simulink model "Model"  (R2024b)
settings: Solver=VariableStepAuto  StartTime=0.0  StopTime=20  RelTol=1e-2
values from neighbouring files (symbols this model uses):
  camber = 1 *pi/180    (= 0.0174532925199)    [var.m]
  cgToRearAxle = 0.7    [var.m]
  cgVerticalToAxlePlane = 0.1    [var.m]
  lammux = 0.65    [var.m]
  lammuy = 0.65    [var.m]
  mass = 200    [var.m]
  maxBrakePressure = 5000000    [var.m]
  tirePressure = 83000    [var.m]
  tireRadius = 0.2057    [var.m]
  trackWidth = 1    [var.m]
  wheelAngleLimit = 45 *pi/180    (= 0.785398163397)    [var.m]
  yawPolarInertia = 200    [var.m]
undefined symbols (not defined in the file or in its folder): SteerLim, Ts, VEH
libraries: sim3dlib x4, autolibsharedcoupling x2, sim3dautolib x2, vehdynlibviscommon x2, simulink x1, autolibshared x1, autolibshareddiff x1, autolibmappedmotor x1, vehdynlibdriver x1, vehdynlibsteering x1, vehdynlibtire x1, vehdynlibsuspension x1
(part 3 of 3)

== system Model/Visualization/3D Visualization/Enabled/3D Visualization/Ground Following/Annotations/Enabled/Determine Angles In UE Vehicle Body Frame ==
  WheelYaw : Inport
  Fx : Inport  Port=2
  Fy : Inport  Port=3
  Add : Sum
  Add1 : Sum
  Constant1 : Constant  Value=0
  Constant11 : Constant  Value=[zeros(4,1)]
  Constant12 : Constant  Value=[zeros(4,1); ones(4,1).*pi/2]
  Constant2 : Constant  Value=pi
  Constant3 : Constant  Value=[zeros(8,2)]
  Constant4 : Constant  Value=[zeros(12,2)]
  Constant6 : Constant  Value=repmat([0 pi/2 0],[4,1])
  Matrix Concatenate : Concatenate  Mode=Multidimensional array
  Matrix Concatenate1 : Concatenate  Mode=Multidimensional array  ConcatenateDimension=2
  Matrix Concatenate2 : Concatenate  Mode=Multidimensional array
  Matrix Concatenate3 : Concatenate  NumInputs=3  Mode=Multidimensional array
  Matrix Concatenate4 : Concatenate  Mode=Multidimensional array  ConcatenateDimension=2
  Switch8 : Switch  ZeroCross=off  SaturateOnIntegerOverflow=off  InputSameDT=off
  Rotation : Outport
  wires:
  Constant2/1 -> Switch8/1
  Matrix Concatenate2/1 -> Switch8/2
  Constant1/1 -> Switch8/3
  Constant3/1 -> Matrix Concatenate1/1
  Matrix Concatenate1/1 -> Matrix Concatenate/1
  Switch8/1 -> Add/1
  Constant6/1 -> Matrix Concatenate/2
  Fx/1 -> Matrix Concatenate2/1
  Fy/1 -> Matrix Concatenate2/2
  Add/1 -> Matrix Concatenate1/2
  Constant12/1 -> Add/2
  Constant11/1 -> Matrix Concatenate3/3
  WheelYaw/1 -> Matrix Concatenate3/1, Matrix Concatenate3/2
  Constant4/1 -> Matrix Concatenate4/1
  Matrix Concatenate3/1 -> Matrix Concatenate4/2
  Matrix Concatenate4/1 -> Add1/2
  Matrix Concatenate/1 -> Add1/1
  Add1/1 -> Rotation/1

== system Model/Visualization/3D Visualization/Enabled/3D Visualization/Physical Vehicle/Annotations/Enabled/Convert to string ==
  xdot : Inport
  MotorSpeed : Inport  Port=2
  Gear : Inport  Port=3
  Round : Rounding  Operator=round
  Round1 : Rounding  Operator=round
  Signal Specification : SignalSpecification  Unit=rpm
  Signal Specification1 : SignalSpecification  Unit=km/h
  String Concatenate1 : StringConcatenate  Inputs=3
  String Concatenate2 : StringConcatenate
  String Concatenate3 : StringConcatenate
  String Constant3 : StringConstant  String="\" km/h\\n\""
  String Constant4 : StringConstant  String="\" RPM\\n\""
  To String1 : ToString
  To String2 : ToString
  To String3 : ToString
  Unit Conversion : UnitConversion
  Unit Conversion1 : UnitConversion
  String : Outport
  wires:
  MotorSpeed/1 -> Unit Conversion/1
  Signal Specification/1 -> Round1/1
  String Constant4/1 -> String Concatenate3/2
  Signal Specification1/1 -> Round/1
  String Concatenate2/1 -> String Concatenate1/1
  To String2/1 -> String Concatenate2/1
  String Constant3/1 -> String Concatenate2/2
  To String1/1 -> String Concatenate1/3
  String Concatenate3/1 -> String Concatenate1/2
  To String3/1 -> String Concatenate3/1
  Round/1 -> To String2/1
  Round1/1 -> To String3/1
  String Concatenate1/1 -> String/1
  Gear/1 -> To String1/1
  Unit Conversion/1 -> Signal Specification/1
  Unit Conversion1/1 -> Signal Specification1/1
  xdot/1 -> Unit Conversion1/1

== system Model/Visualization/3D Visualization/Enabled/3D Visualization/Physical Vehicle/Annotations/Enabled/Determine Angles In UE Vehicle Body Frame ==
  WheelYaw : Inport
  Fx : Inport  Port=2
  Fy : Inport  Port=3
  Add : Sum
  Add1 : Sum
  Constant1 : Constant  Value=0
  Constant11 : Constant  Value=[zeros(4,1)]
  Constant12 : Constant  Value=[zeros(4,1); ones(4,1).*pi/2]
  Constant2 : Constant  Value=pi
  Constant3 : Constant  Value=[zeros(8,2)]
  Constant4 : Constant  Value=[zeros(12,2)]
  Constant6 : Constant  Value=repmat([0 pi/2 0],[4,1])
  Matrix Concatenate : Concatenate  Mode=Multidimensional array
  Matrix Concatenate1 : Concatenate  Mode=Multidimensional array  ConcatenateDimension=2
  Matrix Concatenate2 : Concatenate  Mode=Multidimensional array
  Matrix Concatenate3 : Concatenate  NumInputs=3  Mode=Multidimensional array
  Matrix Concatenate4 : Concatenate  Mode=Multidimensional array  ConcatenateDimension=2
  Switch8 : Switch  ZeroCross=off  SaturateOnIntegerOverflow=off  InputSameDT=off
  Rotation : Outport
  wires:
  Constant2/1 -> Switch8/1
  Matrix Concatenate2/1 -> Switch8/2
  Constant1/1 -> Switch8/3
  Constant3/1 -> Matrix Concatenate1/1
  Matrix Concatenate1/1 -> Matrix Concatenate/1
  Switch8/1 -> Add/1
  Constant6/1 -> Matrix Concatenate/2
  Fx/1 -> Matrix Concatenate2/1
  Fy/1 -> Matrix Concatenate2/2
  Add/1 -> Matrix Concatenate1/2
  Constant12/1 -> Add/2
  Constant11/1 -> Matrix Concatenate3/3
  WheelYaw/1 -> Matrix Concatenate3/1, Matrix Concatenate3/2
  Constant4/1 -> Matrix Concatenate4/1
  Matrix Concatenate3/1 -> Matrix Concatenate4/2
  Matrix Concatenate4/1 -> Add1/2
  Matrix Concatenate/1 -> Add1/1
  Add1/1 -> Rotation/1

== system Model/Visualization/3D Visualization/Enabled/3D Visualization/Simulation 3D Vehicle/Annotations/Enabled/Convert to string ==
  xdot : Inport
  MotorSpeed : Inport  Port=2
  Gear : Inport  Port=3
  Max : MinMax  Function=max  ZeroCross=off
  Round : Rounding  Operator=round
  Round1 : Rounding  Operator=round
  Signal Specification : SignalSpecification  Unit=rpm
  Signal Specification1 : SignalSpecification  Unit=km/h
  String Concatenate1 : StringConcatenate  Inputs=3
  String Concatenate2 : StringConcatenate
  String Concatenate3 : StringConcatenate
  String Constant3 : StringConstant  String="\" km/h\\n\""
  String Constant4 : StringConstant  String="\" RPM\\n\""
  To String1 : ToString
  To String2 : ToString
  To String3 : ToString
  Unit Conversion : UnitConversion
  Unit Conversion1 : UnitConversion
  String : Outport
  wires:
  MotorSpeed/1 -> Unit Conversion/1
  Signal Specification/1 -> Round1/1
  String Constant4/1 -> String Concatenate3/2
  Signal Specification1/1 -> Round/1
  String Concatenate2/1 -> String Concatenate1/1
  To String2/1 -> String Concatenate2/1
  String Constant3/1 -> String Concatenate2/2
  To String1/1 -> String Concatenate1/3
  String Concatenate3/1 -> String Concatenate1/2
  To String3/1 -> String Concatenate3/1
  Round/1 -> To String2/1
  Round1/1 -> Max/1
  String Concatenate1/1 -> String/1
  Gear/1 -> To String1/1
  Unit Conversion/1 -> Signal Specification/1
  Unit Conversion1/1 -> Signal Specification1/1
  xdot/1 -> Unit Conversion1/1
  Max/1 -> To String3/1

== system Model/Visualization/3D Visualization/Enabled/3D Visualization/Simulation 3D Vehicle/Annotations/Enabled/Determine Angles In UE Vehicle Body Frame ==
  WheelYaw : Inport
  Fx : Inport  Port=2
  Fy : Inport  Port=3
  Add : Sum
  Add1 : Sum
  Constant1 : Constant  Value=0
  Constant11 : Constant  Value=[zeros(4,1)]
  Constant12 : Constant  Value=[zeros(4,1); ones(4,1).*pi/2]
  Constant2 : Constant  Value=pi
  Constant3 : Constant  Value=[zeros(8,2)]
  Constant4 : Constant  Value=[zeros(12,2)]
  Constant6 : Constant  Value=repmat([0 pi/2 0],[4,1])
  Matrix Concatenate : Concatenate  Mode=Multidimensional array
  Matrix Concatenate1 : Concatenate  Mode=Multidimensional array  ConcatenateDimension=2
  Matrix Concatenate2 : Concatenate  Mode=Multidimensional array
  Matrix Concatenate3 : Concatenate  NumInputs=3  Mode=Multidimensional array
  Matrix Concatenate4 : Concatenate  Mode=Multidimensional array  ConcatenateDimension=2
  Switch8 : Switch  ZeroCross=off  SaturateOnIntegerOverflow=off  InputSameDT=off
  Rotation : Outport
  wires:
  Constant2/1 -> Switch8/1
  Matrix Concatenate2/1 -> Switch8/2
  Constant1/1 -> Switch8/3
  Constant3/1 -> Matrix Concatenate1/1
  Matrix Concatenate1/1 -> Matrix Concatenate/1
  Switch8/1 -> Add/1
  Constant6/1 -> Matrix Concatenate/2
  Fx/1 -> Matrix Concatenate2/1
  Fy/1 -> Matrix Concatenate2/2
  Add/1 -> Matrix Concatenate1/2
  Constant12/1 -> Add/2
  Constant11/1 -> Matrix Concatenate3/3
  WheelYaw/1 -> Matrix Concatenate3/1, Matrix Concatenate3/2
  Constant4/1 -> Matrix Concatenate4/1
  Matrix Concatenate3/1 -> Matrix Concatenate4/2
  Matrix Concatenate4/1 -> Add1/2
  Matrix Concatenate/1 -> Add1/1
  Add1/1 -> Rotation/1

== matlab function Model/Vehicle Velocity to Wheel Velocity Vectors/Vehicle Velocity to Wheel Velocity Vectors ==
  data: whlAng input; Vx output; vehVel input; Vy output
function [Vx,Vy] = fcn(whlAng, vehVel)
Vx = zeros(4,1);
Vy = zeros(4,1);

for i = 1:4
    a = whlAng(i);
    V = [cos(-a) -sin(-a); sin(-a) cos(-a)] * vehVel;
    Vx(i) = V(1);
    Vy(i) = V(2);
end
